simulink model "SLC"  (R2026a)
settings: Solver=FixedStepAuto  StopTime=20  FixedStep=0.01  EnableMultiTasking=on
undefined symbols (not defined in the file): slc_Ki, slc_Kp, slc_low_sat, slc_up_sat, T_peak, Ts
libraries: simulink x3, slpidlib x1
settings Model: Creator=Utente  LastModifiedBy=zinga
settings OptimizationCC: DefaultUnderspecifiedDataType=single
settings HardwareCC: ProdLargestAtomicInteger=Long  ProdLargestAtomicFloat=Double  ProdHWDeviceType=ARM Compatible->ARM Cortex-M
settings RTWCC: SystemTargetFile=ert.tlc  DataTypeReplacement=CDataTypesFixedWidth  Description=Embedded Coder
settings ERTTargetCC: EnableUserReplacementTypes=on  MaxIdInt64=INT64_MAX  MinIdInt64=INT64_MIN  MaxIdUint64=UINT64_MAX  MaxIdInt32=INT32_MAX  MinIdInt32=INT32_MIN  MaxIdUint32=UINT32_MAX  MaxIdInt16=INT16_MAX  MinIdInt16=INT16_MIN  MaxIdUint16=UINT16_MAX  MaxIdInt8=INT8_MAX  MinIdInt8=INT8_MIN  MaxIdUint8=UINT8_MAX  GenerateSampleERTMain=on  CodeInterfacePackaging=Reusable function

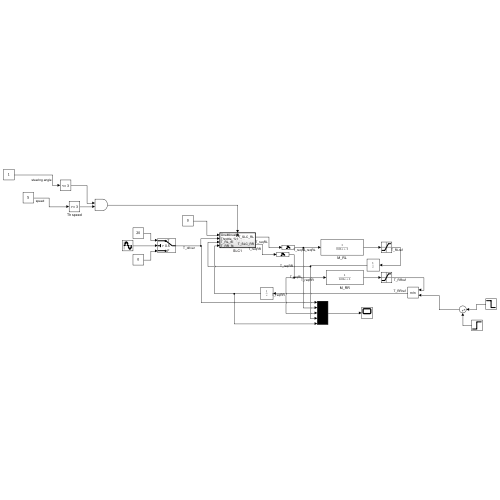
[thumbnail: Simulink's stored preview of the top-level diagram]
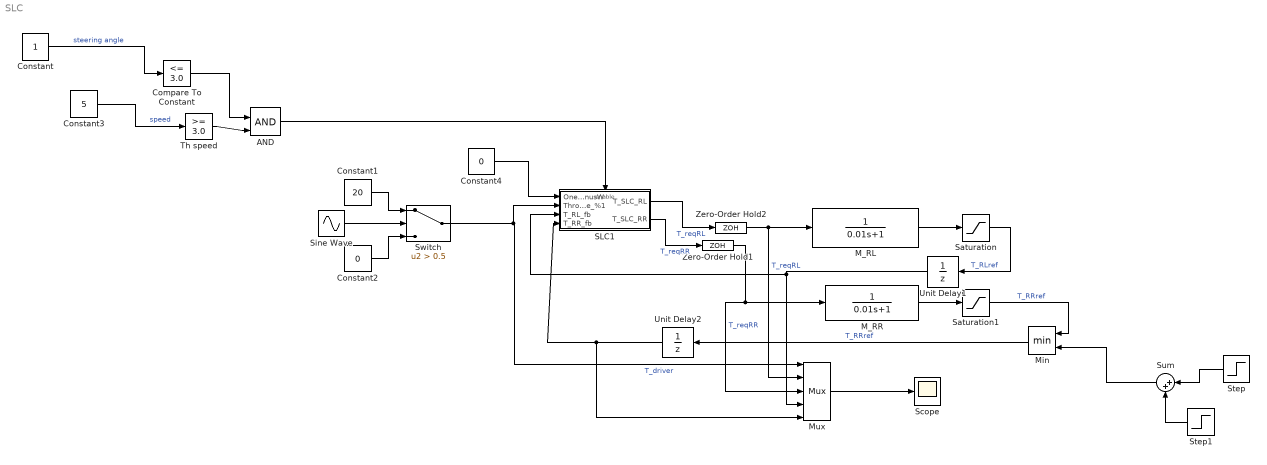
== system SLC ==
  AND : Logic  IconShape=distinctive  AllPortsSameDT=off  OutDataTypeStr=boolean
  Compare To Constant : simulink/Logic and Bit Operations/Compare To Constant  relop=<=  const=3.0  OutDataTypeStr=boolean
  Constant : Constant
  Constant1 : Constant  Value=20
  Constant2 : Constant  Value=0
  Constant3 : Constant  Value=5
  Constant4 : Constant  Value=0
  M_RL : TransferFcn  Denominator=[0.01 1]
  M_RR : TransferFcn  Denominator=[0.01 1]
  Min : MinMax  Inputs=2
  Mux : Mux  Inputs=5
  SLC1 : Subsystem  TreatAsAtomicUnit=on
  Saturation : Saturate  UpperLimit=21  LowerLimit=-21
  Saturation1 : Saturate  UpperLimit=21  LowerLimit=-21
  Scope : Scope
      settings: ActiveDisplayYMinimum=1.4080718802065189  ActiveDisplayYMaximum=18.911191161536266
  Sine Wave : Sin  Frequency=0.2  SampleTime=0.01
  Step : Step  Time=3  InitialValue=21  FinalValue=8  SampleTime=0
  Step1 : Step  Time=9  FinalValue=13  SampleTime=0
  Sum : Sum  Inputs=|++
  Switch : Switch  Criteria=u2 > Threshold  Threshold=0.5  SaturateOnIntegerOverflow=off  InputSameDT=off
  Th speed : simulink/Logic and Bit Operations/Compare To Constant  relop=>=  const=3.0  OutDataTypeStr=boolean
  Unit Delay1 : UnitDelay  SampleTime=-1
  Unit Delay2 : UnitDelay  SampleTime=-1
  Zero-Order Hold1 : ZeroOrderHold  SampleTime=0.01
  Zero-Order Hold2 : ZeroOrderHold  SampleTime=0.01
  wires:
  Compare To Constant/1 -> AND/1
  Constant/1 -> Compare To Constant/1  "steering angle"
  SLC1/1(T_SLC_RL) -> Zero-Order Hold2/1  "T_reqRL"
  SLC1/2(T_SLC_RR) -> Zero-Order Hold1/1  "T_reqRR"
  Mux/1 -> Scope/1
  M_RL/1 -> Saturation/1
  Saturation/1 -> Unit Delay1/1  "T_RLref"
  Sine Wave/1 -> Switch/2
  Constant1/1 -> Switch/1
  Constant2/1 -> Switch/3
  Switch/1 -> SLC1/2(Throttle_%1), Mux/1  "T_driver"
  M_RR/1 -> Saturation1/1
  Min/1 -> Unit Delay2/1  "T_RRref"
  Constant3/1 -> Th speed/1  "speed"
  Th speed/1 -> AND/2
  AND/1 -> SLC1/Enable
  Saturation1/1 -> Min/1  "T_RRref"
  Step/1 -> Sum/1
  Sum/1 -> Min/2
  Step1/1 -> Sum/2
  Unit Delay1/1 -> SLC1/3(T_RL_fb), Mux/4
  Unit Delay2/1 -> SLC1/4(T_RR_fb), Mux/5
  Zero-Order Hold1/1 -> Mux/3, M_RR/1  "T_reqRR"
  Zero-Order Hold2/1 -> Mux/2, M_RL/1  "T_reqRL"
  Constant4/1 -> SLC1/1(OneMinusW)

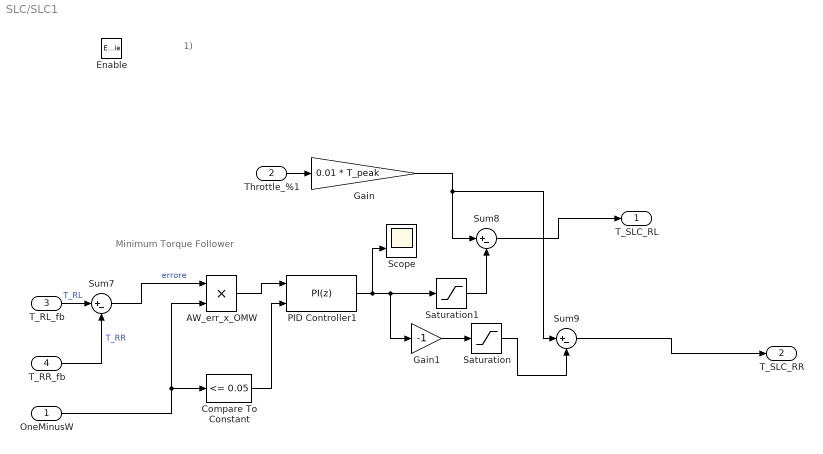
== system SLC/SLC1 ==
  note: 1)
  note: Minimum Torque Follower
  OneMinusW : Inport
  Throttle_%1 : Inport  Port=2
  T_RL_fb : Inport  Port=3
  T_RR_fb : Inport  Port=4
  Enable : EnablePort
  AW_err_x_OMW : Product  Inputs=**
  Compare To Constant : simulink/Logic and Bit Operations/Compare To Constant  relop=<=  const=0.05  OutDataTypeStr=boolean
  Gain : Gain  Gain=0.01 * T_peak
  Gain1 : Gain  Gain=-1
  PID Controller1 : slpidlib/PID Controller  Controller=PI  Form=Parallel  TimeDomain=Discrete-time  UseExternalTs=off  SampleTime=Ts  IntegratorMethod=Forward Euler  FilterMethod=Forward Euler  ControllerParametersSource=internal  P=slc_Kp  I=slc_Ki  UseKiTs=off  D=0  UseExternalDerivativeSource=off  N=100  UseFilter=off  TunerSelectOption=Transfer Function Based (PID Tuner App)  InitialConditionSource=internal  InitialConditionForIntegrator=0  InitialConditionForFilter=0  DifferentiatorICPrevScaledInput=0  ExternalReset=level  TrackingMode=off  Kt=1  LimitOutput=on  SatLimitsSource=internal  UpperSaturationLimit=slc_up_sat  LowerSaturationLimit=slc_low_sat  LinearizeAsGain=on  AntiWindupMode=back-calculation  Kb=1  LimitIntegrator=off  UpperIntegratorSaturationLimit=inf  LowerIntegratorSaturationLimit=-inf  POutMin=[]  POutMax=[]  IOutMin=[]  IOutMax=[]  DOutMin=[]  DOutMax=[]  NOutMin=[]  NOutMax=[]  SumOutMin=[]  SumOutMax=[]  SaturationOutMin=[]  SaturationOutMax=[]  PParamMin=[]  PParamMax=[]  IParamMin=[]  IParamMax=[]  DParamMin=[]  DParamMax=[]  NParamMin=[]  NParamMax=[]  KbParamMin=[]  KbParamMax=[]  KtParamMin=[]  KtParamMax=[]  KbOutMin=[]  KbOutMax=[]  KtOutMin=[]  KtOutMax=[]  IntegratorOutMin=[]  IntegratorOutMax=[]  FilterOutMin=[]  FilterOutMax=[]  SumI1OutMin=[]  SumI1OutMax=[]  SumI2OutMin=[]  SumI2OutMax=[]  SumI3OutMin=[]  SumI3OutMax=[]  SumI4OutMin=[]  SumI4OutMax=[]  SumDOutMin=[]  SumDOutMax=[]  DifferentiatorOutMin=[]  DifferentiatorOutMax=[]  FilterDiffOutCoefMin=[]  FilterDiffOutCoefMax=[]  ReciprocalOutMin=[]  ReciprocalOutMax=[]  SumDenOutMin=[]  SumDenOutMax=[]  SumNumOutMin=[]  SumNumOutMax=[]  DivideOutMin=[]  DivideOutMax=[]  UdiffTsProdOutMin=[]  UdiffTsProdOutMax=[]  NTsProdOutMin=[]  NTsProdOutMax=[]  UintegralTsProdOutMin=[]  UintegralTsProdOutMax=[]  UngainTsProdOutMin=[]  UngainTsProdOutMax=[]  ClampingZeroOutDataTypeStr=Inherit: Inherit via back propagation  ClampingZeroOutMin=[]  ClampingZeroOutMax=[]  FilterDenConstantOutDataTypeStr=Inherit: Inherit via back propagation  FilterDenConstantOutMin=[]  FilterDenConstantOutMax=[]  PCopyOutDataTypeStr=Inherit: Inherit via back propagation  PCopyOutMin=[]  PCopyOutMax=[]  NCopyOutDataTypeStr=Inherit: Inherit via back propagation  NCopyOutMin=[]  NCopyOutMax=[]  IntegratorContinuousStateAttributes=''  IntegratorStateMustResolveToSignalObject=off  IntegratorRTWStateStorageClass=Auto  FilterContinuousStateAttributes=''  FilterStateMustResolveToSignalObject=off  FilterRTWStateStorageClass=Auto  ParallelPVariant=InternalParameters  IdealPVariant=Disabled  IVariant=InternalParameters  DVariant=Disabled  IntegratorVariant=Discrete  SatVariant=Enabled  AWVariant=BackCalculation  PCopyVariant=Disabled  TRVariant=Disabled  FdbkBlocksVariant=Forward  IdealPFdbkVariant=Disabled  SatFdbkVariant=Disabled  DerivativeFilterVariant=Disabled  NVariant=Disabled  NCopyVariant=Disabled_SignalSpec  FilterICVariant=Disabled  IntegratorICVariant=InternalICs  ExternalResetVariant=ExternalReset  TRSumVariant=Passthrough  SumFdbkVariant=Disabled  SumVariant=Sum_PI  TsampFilterVariant=InternalTs  TsampNgainVariant=Passthrough  TsampIntegralVariant=Disabled_SignalSpec  ExternalSaturationOutDataTypeStr=Inherit: Same as second input  DerivativeSourceVariant=Disabled  PreIntVariant=InternalPreInt
  Saturation : Saturate  UpperLimit=inf  LowerLimit=0
  Saturation1 : Saturate  UpperLimit=inf  LowerLimit=0
  Scope : Scope  NumInputPorts=2
      settings: ActiveDisplayYMinimum=-14.980593372573752  ActiveDisplayYMaximum=14.997843708063737
  Sum7 : Sum  Inputs=|+-
  Sum8 : Sum  Inputs=|+-
  Sum9 : Sum  Inputs=|+-
  T_SLC_RL : Outport
  T_SLC_RR : Outport  Port=2
  wires:
  PID Controller1/1 -> Saturation1/1, Gain1/1, Scope/2
  Gain/1 -> Sum8/1, Sum9/1
  Sum8/1 -> T_SLC_RL/1
  T_RR_fb/1 -> Sum7/2  "T_RR"
  Saturation1/1 -> Sum8/2
  Gain1/1 -> Saturation/1
  Sum9/1 -> T_SLC_RR/1
  Throttle_%1/1 -> Gain/1
  OneMinusW/1 -> Compare To Constant/1, AW_err_x_OMW/2
  Compare To Constant/1 -> PID Controller1/2
  Saturation/1 -> Sum9/2
  AW_err_x_OMW/1 -> PID Controller1/1
  Sum7/1 -> AW_err_x_OMW/1  "errore"
  T_RL_fb/1 -> Sum7/1  "T_RL"
